simulink model "Solar_Seguidor"  (R2021b)
settings: Solver=ode1  StartTime=0.0  StopTime=inf  FixedStep=25e-6  RelTol=1e-3
PostLoadFcn:
  | %clc; clear all; close all;
  | %%%%%%%%%%%%%%%%%%%%%%%%%%%%%%%%%%%%%%%%%%%%%%%%
  | %%%%%%%%% Solar seguidor de rede %%%%%%%%%%
  | %%%%%%%%%%%%%%%%%%%%%%%%%%%%%%%%%%%%%%%%%%%%%%%%
  | %%%% Nominal Parameters %%%%
  | Pnom = 16e3;                                         % Potencia Nominal
  | Vnom_rms = 210;                                    % V linha rms
  | Vnom_peak = sqrt(2/3)*Vnom_rms;                     % V fase pico
  | FP_min = 1;                                       % Para suporte de reativo
  | Snom = Pnom/FP_min;                                 % Potencia aparente
  | Irms = Pnom/(sqrt(3)*Vnom_rms);                     % Ig rms
  | Inom_peak = Irms*sqrt(2);                           % Ig pico
  | Zbase = Vnom_peak/Inom_peak;                        % Impedancia Base
  | f = 60;                                             % Freq nominal
  | wnom = 2*pi*60;                                     % Freq Ang. nominal
  | m = 0.805;                                            % Indice mod nominal
  | Vdc = 2*(Vnom_peak/m);                              % Vcc
  | Vdc_2 = Vdc/2;                                      % Metade Vcc
  | Kconv = Zbase;                                      % Ganho conversor
  | %%%% Transformer %%%%
  | S_trafo = 250e3;                                      % transformer apparent power
  | Vrms_high = 400;                                   % transformer secondary voltage - Wye connection
  | Vrms_low = 210;                                   % transformer primary voltage - Delta connection
  | N = Vrms_high/Vrms_low;                             % transformation relationship
  | X_pu_trafo = 0.03;                                 % transformer p.u. reactance
  | Zb_trafo_high = ((Vrms_high)^2)/S_trafo;            % secondary base impedance
  | Zb_trafo = ((Vnom_rms)^2)/S_trafo;                  % primary base impedance
  | L_trafo = (X_pu_trafo*Zb_trafo)/wnom;               % primary inductance
  | %%%% LCL Filter Project %%%%
  | fsw = 105*60;%105*60;                                         % switching frequency
  | ripple = 0.05;                                       % current ripple
  | L1 = Vdc/(6*ripple*Inom_peak*fsw);                  % inductor L1
  |  RL1 = 0.005;                                        % L1 resistance
  |  Cbase = 1/(wnom*Kconv);                             % base capacitance
  |  Cf = 0.05*Cbase;                                    % filter capacitor
  | % Calculo do filtro
  | Sbase = 16e3;
  | %Sbase = 200e3*1.12;
  | V_LL = 210;
  | V_LG = 210/sqrt(3);
  | Vbase = V_LG*sqrt(2);
  | Ibase = (Sbase*sqrt(2))/(V_LG*3)*sqrt(3/2);
  | Zbase = (V_LL^2)/Sbase;
  | Rbase = Zbase;
  | Xbase = Zbase;
  | Lbase = Xbase/(2*pi*60);
  | Cbase = 1/(Xbase*2*pi*60);
  | w = 2*pi*60;
  | Q = 70;
  | Lf = 0.15*Lbase;
  | Cf = 0.05*Cbase;
  | fc = 1/(2*pi*sqrt(Lf*Cf));
  | R = (w*Lf)/Q;
  | Lf = L1;
  | R = RL1;
  | ka=0.2;                                             % attenuation factor
  | L2 = (sqrt(1/(ka^2))+1)/(Cf*((2*pi*fsw)^2));        % inductor L2
  | RL2 = 0.005;                                        % L2 resistance
  | w_res = sqrt((L1+L2+L_trafo)/(L1*L2*Cf));           % resonant angular frequency
  | f_res = w_res/(2*pi);                               % resonant frequency
  | Rf = 1/(3*w_res*Cf);                                % filter capacitor resistance
  | %%%%%%%%%%%%%%%%%%%%%%%%
  | %%%% Control Design %%%%
  | %%%%%%%%%%%%%%%%%%%%%%%%
  | %%%% Power Control %%%%
  | Ron = 0.0001;
  | tau_i = 0.5e-3;                                       % tempo de resposta
  | kp_current = (Lf+L_trafo)/tau_i;
  | ki_current = (R+Ron)/tau_i;
  | decouple = (wnom*Lf);
  | kp_current_pu = kp_current/Kconv;                  % Adaptando para pu
  | ki_current_pu = ki_current/Kconv;
  | decouple_pu = (wnom*Lf+(R+Ron))/Kconv;
  | %%%% Dc Link Control %%%%
  | Iext = Pnom/Vdc;
  | Kcc = Vdc/Iext;
  | Sbase = 16e3;
  | C_cc_proj = (Sbase/(2*pi*60*Vdc*Vdc*0.05));
  | 
  | % Controle de tensao
  | a = 3;
  | kp_dc = (C_cc_proj)/(2*a*tau_i);
  | ti_dc = (a^2)*tau_i;
  | ki_dc = kp_dc/ti_dc;
  | kp_dc_pu = (Kcc*C_cc_proj)/(2*a*tau_i);
  | ki_dc_pu = kp_dc_pu/ti_dc;
  | 
  | Ts = 25e-6;
  | 
  | 
  |  Ts_Control=2*Ts;Ts_Power=Ts;
InitFcn:
  | %clc; clear all; close all;
  | %%%%%%%%%%%%%%%%%%%%%%%%%%%%%%%%%%%%%%%%%%%%%%%%
  | %%%%%%%%% Solar seguidor de rede %%%%%%%%%%
  | %%%%%%%%%%%%%%%%%%%%%%%%%%%%%%%%%%%%%%%%%%%%%%%%
  | %%%% Nominal Parameters %%%%
  | Pnom = 16e3;                                         % Potencia Nominal
  | Vnom_rms = 210;                                    % V linha rms
  | Vnom_peak = sqrt(2/3)*Vnom_rms;                     % V fase pico
  | FP_min = 1;                                       % Para suporte de reativo
  | Snom = Pnom/FP_min;                                 % Potencia aparente
  | Irms = Pnom/(sqrt(3)*Vnom_rms);                     % Ig rms
  | Inom_peak = Irms*sqrt(2);                           % Ig pico
  | Zbase = Vnom_peak/Inom_peak;                        % Impedancia Base
  | f = 60;                                             % Freq nominal
  | wnom = 2*pi*60;                                     % Freq Ang. nominal
  | m = 0.805;                                            % Indice mod nominal
  | Vdc = 2*(Vnom_peak/m);                              % Vcc
  | Vdc_2 = Vdc/2;                                      % Metade Vcc
  | Kconv = Zbase;                                      % Ganho conversor
  | %%%% Transformer %%%%
  | S_trafo = 250e3;                                      % transformer apparent power
  | Vrms_high = 400;                                   % transformer secondary voltage - Wye connection
  | Vrms_low = 210;                                   % transformer primary voltage - Delta connection
  | N = Vrms_high/Vrms_low;                             % transformation relationship
  | X_pu_trafo = 0.03;                                 % transformer p.u. reactance
  | Zb_trafo_high = ((Vrms_high)^2)/S_trafo;            % secondary base impedance
  | Zb_trafo = ((Vnom_rms)^2)/S_trafo;                  % primary base impedance
  | L_trafo = (X_pu_trafo*Zb_trafo)/wnom;               % primary inductance
  | %%%% LCL Filter Project %%%%
  | fsw = 105*60;%105*60;                                         % switching frequency
  | ripple = 0.05;                                       % current ripple
  | L1 = Vdc/(6*ripple*Inom_peak*fsw);                  % inductor L1
  |  RL1 = 0.005;                                        % L1 resistance
  |  Cbase = 1/(wnom*Kconv);                             % base capacitance
  |  Cf = 0.05*Cbase;                                    % filter capacitor
  | % Calculo do filtro
  | Sbase = 16e3;
  | %Sbase = 200e3*1.12;
  | V_LL = 210;
  | V_LG = 210/sqrt(3);
  | Vbase = V_LG*sqrt(2);
  | Ibase = (Sbase*sqrt(2))/(V_LG*3)*sqrt(3/2);
  | Zbase = (V_LL^2)/Sbase;
  | Rbase = Zbase;
  | Xbase = Zbase;
  | Lbase = Xbase/(2*pi*60);
  | Cbase = 1/(Xbase*2*pi*60);
  | w = 2*pi*60;
  | Q = 70;
  | Lf = 0.15*Lbase;
  | Cf = 0.05*Cbase;
  | fc = 1/(2*pi*sqrt(Lf*Cf));
  | R = (w*Lf)/Q;
  | Lf = L1;
  | R = RL1;
  | ka=0.2;                                             % attenuation factor
  | L2 = (sqrt(1/(ka^2))+1)/(Cf*((2*pi*fsw)^2));        % inductor L2
  | RL2 = 0.005;                                        % L2 resistance
  | w_res = sqrt((L1+L2+L_trafo)/(L1*L2*Cf));           % resonant angular frequency
  | f_res = w_res/(2*pi);                               % resonant frequency
  | Rf = 1/(3*w_res*Cf);                                % filter capacitor resistance
  | %%%%%%%%%%%%%%%%%%%%%%%%
  | %%%% Control Design %%%%
  | %%%%%%%%%%%%%%%%%%%%%%%%
  | %%%% Power Control %%%%
  | Ron = 0.0001;
  | tau_i = 0.5e-3;                                       % tempo de resposta
  | kp_current = (Lf+L_trafo)/tau_i;
  | ki_current = (R+Ron)/tau_i;
  | decouple = (wnom*Lf);
  | kp_current_pu = kp_current/Kconv;                  % Adaptando para pu
  | ki_current_pu = ki_current/Kconv;
  | decouple_pu = (wnom*Lf+(R+Ron))/Kconv;
  | %%%% Dc Link Control %%%%
  | Iext = Pnom/Vdc;
  | Kcc = Vdc/Iext;
  | Sbase = 16e3;
  | C_cc_proj = (Sbase/(2*pi*60*Vdc*Vdc*0.05));
  | 
  | % Controle de tensao
  | a = 3;
  | kp_dc = (C_cc_proj)/(2*a*tau_i);
  | ti_dc = (a^2)*tau_i;
  | ki_dc = kp_dc/ti_dc;
  | kp_dc_pu = (Kcc*C_cc_proj)/(2*a*tau_i);
  | ki_dc_pu = kp_dc_pu/ti_dc;
  | 
  | Ts = 25e-6;
  | 
  | 
  |  Ts_Control=2*Ts;Ts_Power=Ts;
undefined symbols (not defined in the file): D1, Delta, DIN_2A_Ch00, DiscIntNeverNeededParam, eHS, I, Kp_dc, Left, parameter_set_id, ph, signal1, signal2, signal3, signal4, signal5, signal6, signal7, type, V
libraries: rtlab x11, spsCurrentMeasurementLib x4, spsabctodq0Lib x4, spsThreePhaseVIMeasurementLib x3, spsThreePhaseSeriesRLCBranchLib x3, spsPLL3phLib x3, spsTHDLib x3, artemis x2, spsOnDelayLib x2, spsSeriesRLCBranchLib x2, spsRMSLib x2, slpidlib x2
(part 1 of 2)
settings Model: ARTEMISmethode_block_infos=$$__separator__$$Solar_Seguidor/ARTEMIS Guide1$$__separator__$$  Creator=Lafae  LastModifiedBy=lafae
settings SolverCC: AlgebraicLoopSolver=LineSearch
settings DataIOCC: SaveOutput=off  SaveTime=off  ReturnWorkspaceOutputs=off
settings OptimizationCC: BlockReduction=off  OptimizeBlockIOStorage=off  BufferReuse=off  GlobalBufferReuse=off  ExpressionFolding=off  LocalBlockOutputs=off  OptimizeDataStoreBuffers=off  BusAssignmentInplaceUpdate=off
settings DebuggingCC: AlgebraicLoopMsg=none  MaxConsecutiveZCsMsg=none  MultiTaskDSMMsg=warning  ParameterOverflowMsg=warning  ModelReferenceExtraNoncontSigs=none  SFMachineParentedDataDiag=warning  ArithmeticOperatorsInVariantConditions=warning
settings SFSimCC: CustomCodeUndefinedFunction=UseInterfaceOnly

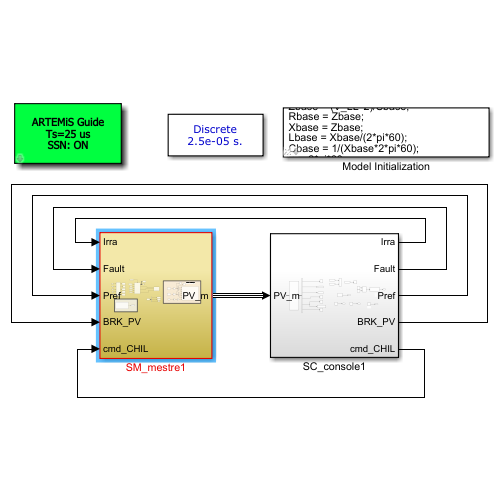
[thumbnail: Simulink's stored preview of the top-level diagram]
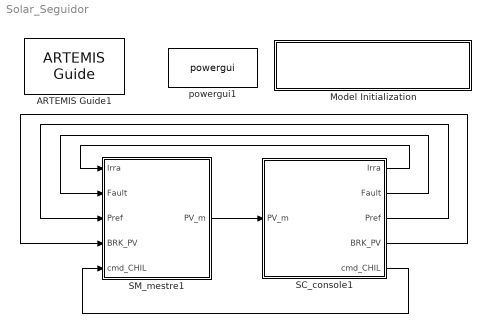
== system Solar_Seguidor ==
  ARTEMIS Guide1 : artemis/ARTEMIS/ARTEMIS Guide  Tag=art7.5  Description=New ARTEMiS block v 7.5b (R2015b+)  lock=on  Ts=Ts  ssn=on  opt=art5  dyna=off  nb_perm=4  RT_fullcomp=off  ssn_itvc=off  ssn_ivic=off  ssn_ext=off  ssn_solver=Art5  iter_type=iSWITCH and iMOV only (default)  ssn_ImpulseLoopBlockedStateUpdate=5  ssn_mov_iter_number=5  ssn_switch_iter_number=3  ssn_lu_or_ldlt=LU (more robust)  ssn_nib_type_verify=on  ssn_use_lu=on  ssn_use_ldlt=off  ssn_impulse=on  ssn_quasimpulse=off  ssn_impulse_loop=5  paraExtinctionThy=off  Thy_Impulse=on  dtc=Off  dtc_opt=normal  ao=off  simtype=off  ct_mac=off  lin_mov=off  lsp=[0.001 2]  spike_skip=Disabled  dtc_extra=1  dtc_sws=normal  dtc_pied=0.5  SPSRulesBlock=SPSRules  tre=off  ctmm=off  LF=off  dpl_type=ARTEMiS DPL  rlc_type=off  custom_type=off  para=on  ssn_full_iteration=off  ssn_init_cond=block only
  Model Initialization : Subsystem  AncestorBlock=artemis/Tools /Misc/Model Initialization  mask(Model Functions){InitFcnX=|, prel=off, posl=on, inif=on, strf=off}
      mask InitFcnX=|
      | %clc; clear all; close all;
      | %%%%%%%%%%%%%%%%%%%%%%%%%%%%%%%%%%%%%%%%%%%%%%%%
      | %%%%%%%%% Solar seguidor de rede %%%%%%%%%%
      | %%%%%%%%%%%%%%%%%%%%%%%%%%%%%%%%%%%%%%%%%%%%%%%%
      | %%%% Nominal Parameters %%%%
      | Pnom = 16e3;                                         % Potencia Nominal
      | Vnom_rms = 210;                                    % V linha rms
      | Vnom_peak = sqrt(2/3)*Vnom_rms;                     % V fase pico
      | FP_min = 1;                                       % Para suporte de reativo
      | Snom = Pnom/FP_min;                                 % Potencia aparente
      | Irms = Pnom/(sqrt(3)*Vnom_rms);                     % Ig rms
      | Inom_peak = Irms*sqrt(2);                           % Ig pico
      | Zbase = Vnom_peak/Inom_peak;                        % Impedancia Base
      | f = 60;                                             % Freq nominal
      | wnom = 2*pi*60;                                     % Freq Ang. nominal
      | m = 0.805;                                            % Indice mod nominal
      | Vdc = 2*(Vnom_peak/m);                              % Vcc
      | Vdc_2 = Vdc/2;                                      % Metade Vcc
      | Kconv = Zbase;                                      % Ganho conversor
      | %%%% Transformer %%%%
      | S_trafo = 250e3;                                      % transformer apparent power
      | Vrms_high = 400;                                   % transformer secondary voltage - Wye connection
      | Vrms_low = 210;                                   % transformer primary voltage - Delta connection
      | N = Vrms_high/Vrms_low;                             % transformation relationship
      | X_pu_trafo = 0.03;                                 % transformer p.u. reactance
      | Zb_trafo_high = ((Vrms_high)^2)/S_trafo;            % secondary base impedance
      | Zb_trafo = ((Vnom_rms)^2)/S_trafo;                  % primary base impedance
      | L_trafo = (X_pu_trafo*Zb_trafo)/wnom;               % primary inductance
      | %%%% LCL Filter Project %%%%
      | fsw = 105*60;%105*60;                                         % switching frequency
      | ripple = 0.05;                                       % current ripple
      | L1 = Vdc/(6*ripple*Inom_peak*fsw);                  % inductor L1
      |  RL1 = 0.005;                                        % L1 resistance
      |  Cbase = 1/(wnom*Kconv);                             % base capacitance
      |  Cf = 0.05*Cbase;                                    % filter capacitor
      | % Calculo do filtro
      | Sbase = 16e3;
      | %Sbase = 200e3*1.12;
      | V_LL = 210;
      | V_LG = 210/sqrt(3);
      | Vbase = V_LG*sqrt(2);
      | Ibase = (Sbase*sqrt(2))/(V_LG*3)*sqrt(3/2);
      | Zbase = (V_LL^2)/Sbase;
      | Rbase = Zbase;
      | Xbase = Zbase;
      | Lbase = Xbase/(2*pi*60);
      | Cbase = 1/(Xbase*2*pi*60);
      | w = 2*pi*60;
      | Q = 70;
      | Lf = 0.15*Lbase;
      | Cf = 0.05*Cbase;
      | fc = 1/(2*pi*sqrt(Lf*Cf));
      | R = (w*Lf)/Q;
      | Lf = L1;
      | R = RL1;
      | ka=0.2;                                             % attenuation factor
      | L2 = (sqrt(1/(ka^2))+1)/(Cf*((2*pi*fsw)^2));        % inductor L2
      | RL2 = 0.005;                                        % L2 resistance
      | w_res = sqrt((L1+L2+L_trafo)/(L1*L2*Cf));           % resonant angular frequency
      | f_res = w_res/(2*pi);                               % resonant frequency
      | Rf = 1/(3*w_res*Cf);                                % filter capacitor resistance
      | %%%%%%%%%%%%%%%%%%%%%%%%
      | %%%% Control Design %%%%
      | %%%%%%%%%%%%%%%%%%%%%%%%
      | %%%% Power Control %%%%
      | Ron = 0.0001;
      | tau_i = 0.5e-3;                                       % tempo de resposta
      | kp_current = (Lf+L_trafo)/tau_i;
      | ki_current = (R+Ron)/tau_i;
      | decouple = (wnom*Lf);
      | kp_current_pu = kp_current/Kconv;                  % Adaptando para pu
      | ki_current_pu = ki_current/Kconv;
      | decouple_pu = (wnom*Lf+(R+Ron))/Kconv;
      | %%%% Dc Link Control %%%%
      | Iext = Pnom/Vdc;
      | Kcc = Vdc/Iext;
      | Sbase = 16e3;
      | C_cc_proj = (Sbase/(2*pi*60*Vdc*Vdc*0.05));
      |
      | % Controle de tensao
      | a = 3;
      | kp_dc = (C_cc_proj)/(2*a*tau_i);
      | ti_dc = (a^2)*tau_i;
      | ki_dc = kp_dc/ti_dc;
      | kp_dc_pu = (Kcc*C_cc_proj)/(2*a*tau_i);
      | ki_dc_pu = kp_dc_pu/ti_dc;
      |
      | Ts = 25e-6;
      |
      |
      |  Ts_Control=2*Ts;Ts_Power=Ts;
      mask prompts: InitFcnX "Initialisation"; prel "Preload Function"; posl "PostLoad Function"; inif "InitFcn"; strf "StartFcn"
      mask init:
      | currentBlock = gcb;
      | root = bdroot(currentBlock);
      | 
      | if ~strcmp(get_param(root,'BlockDiagramType'),'library')
      |     if prel==1
      |         set_param(root, 'PreLoadFcn', InitFcnX);
      |     else
      |         set_param(root, 'PreLoadFcn', '');
      |     end
      |     if inif==1
      |         set_param(root, 'InitFcn', InitFcnX);
      |     else
      |         set_param(root, 'InitFcn', '');
      |     end
      |     if strf==1
      |         set_param(root, 'StartFcn', InitFcnX);
      |     else
      |         set_param(root, 'StartFcn', '');
      |     end
      |     if posl==1
      |         set_param(root, 'PostLoadFcn', InitFcnX);
      |     else
      |         set_param(root, 'PostLoadFcn', '');
      |     end
      | end
      | 
      | pos = get_param(currentBlock, 'Position');
      | width = pos(3) - pos(1); height = pos(4) - pos(2);
      | txt = [ upper(root) '\n' '- InitFcn. . . . . '  get_param(root, 'InitFcn') ];
      settings: CopyFcn=set_param(gcb,'LinkStatus','inactive')
      mask Display: text(5, height*0.5, txt, 'horizontalAlignment', 'left', 'verticalAlignment', 'middle') ;
  SC_console1 : Subsystem
  SM_mestre1 : Subsystem
  powergui1 : spspowerguiLib/powergui  Priority=1  SimulationMode=Discrete  SampleTime=Ts  frequency=60  Iterations=50  frequencyindice=0  Pbase=100e6  ErrMax=1e-4  UnitsV=kV  UnitsW=MW  buscounter=0  FunctionMessages=off  echomessages=off  EnableUseOfTLC=off  CurrentSourceSwitches=off  DisableSnubberDevices=off  DisableRonSwitches=off  DisableVfSwitches=off  DisplayEquations=off  AutomaticDiscreteSolvers=off  SolverType=Tustin/Backward Euler (TBE)  Interpol=off  ExternalGateDelay=off  methode=off  Ts=0  x0status=blocks  SPID=off  SwTol=0  HookPort=off  NonlinearTolerance=0  nMaxIteration=15  ContinueOnMaxIteration=off  RestoreLinks=warning  ResistiveCurrentMeasurement=off  Frange=[0:2:500]  Ylog=off  Xlog=on  ShowGrid=off  save=off  variable=ZData  structure=0  ZoomFFT=on  StartTime=0.0  cycles=1  DisplayStyle=1  fundamental=60  FreqAxis=off  MaxFrequency=1000  frequencyindicesteady=1  RmsSteady=1  display=off
  wires:
  SM_mestre1/1(PV_m) -> SC_console1/1(PV_m)
  SC_console1/1(Irra) -> SM_mestre1/1(Irra)
  SC_console1/2(Fault) -> SM_mestre1/2(Fault)
  SC_console1/3(Pref) -> SM_mestre1/3(Pref)
  SC_console1/4(BRK_PV) -> SM_mestre1/4(BRK_PV)
  SC_console1/5(cmd_CHIL) -> SM_mestre1/5(cmd_CHIL)

== system Solar_Seguidor/Model Initialization ==

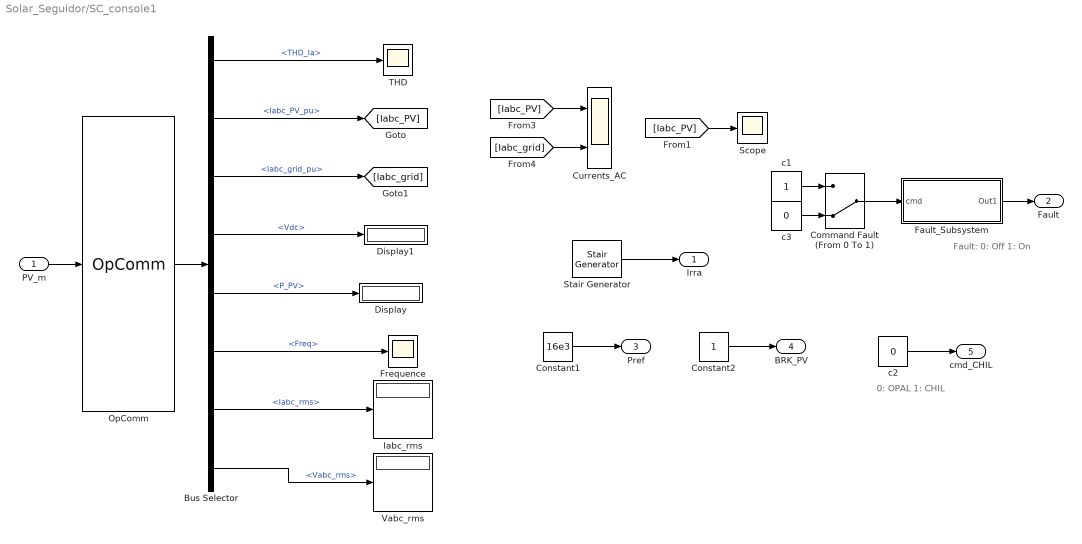
== system Solar_Seguidor/SC_console1 ==
  note: Fault:
      | 0: Off
      | 1: On
  note: 0: OPAL
      | 1: CHIL
  PV_m : Inport
  Bus Selector : BusSelector  OutputSignals=THD_Ia,Iabc_PV_pu,Iabc_grid_pu,Vdc,P_PV,Freq,Iabc_rms,Vabc_rms
  Command Fault (From 0 To 1) : ManualSwitch  CurrentSetting=0
  Constant1 : Constant  Value=16e3
  Constant2 : Constant
  Currents_AC : Scope  NumInputPorts=2
  Display : Display
  Display1 : Display
  Fault_Subsystem : Subsystem
  Frequence : Scope
  Iabc_rms : Display
  OpComm : rtlab/OpComm  nbport=1  groupe_acq=1  subsys_rate=0  st=0  Synchronization=on  Interpolation=on  Threshold=1.0  Missed_Data=off  Sim_Time=off  Samples=off  dynSigOut=off  from_console=0  warning_done=off  writeOpCommFile=off  Offset=off
      settings: SourceProductName=RT-LAB
  Scope : Scope
  Stair Generator : spsStairGeneratorLib/Stair Generator  t=[0, 1, 3, 5,7]  e=[10, 4, 7.5, 10,10]*1e2  Ts=0
  THD : Scope
  Vabc_rms : Display
  c1 : Constant
  c2 : Constant  Value=0
  c3 : Constant  Value=0
  Irra : Outport
  Fault : Outport  Port=2
  Pref : Outport  Port=3
  BRK_PV : Outport  Port=4
  cmd_CHIL : Outport  Port=5
  wires:
  [Iabc_PV] -> Currents_AC/1
  [Iabc_grid] -> Currents_AC/2
  PV_m/1 -> OpComm/1
  Bus Selector/2 -> [Iabc_PV]  "<Iabc_PV_pu>"
  Stair Generator/1 -> Irra/1
  Fault_Subsystem/1(Out1) -> Fault/1
  c1/1 -> Command Fault (From 0 To 1)/1
  c3/1 -> Command Fault (From 0 To 1)/2
  Command Fault (From 0 To 1)/1 -> Fault_Subsystem/1(cmd)
  Constant1/1 -> Pref/1
  [Iabc_PV] -> Scope/1
  OpComm/1 -> Bus Selector/1
  Bus Selector/1 -> THD/1  "<THD_Ia>"
  Bus Selector/3 -> [Iabc_grid]  "<Iabc_grid_pu>"
  Bus Selector/4 -> Display1/1  "<Vdc>"
  Bus Selector/5 -> Display/1  "<P_PV>"
  Bus Selector/6 -> Frequence/1  "<Freq>"
  Constant2/1 -> BRK_PV/1
  c2/1 -> cmd_CHIL/1
  Bus Selector/7 -> Iabc_rms/1  "<Iabc_rms>"
  Bus Selector/8 -> Vabc_rms/1  "<Vabc_rms>"

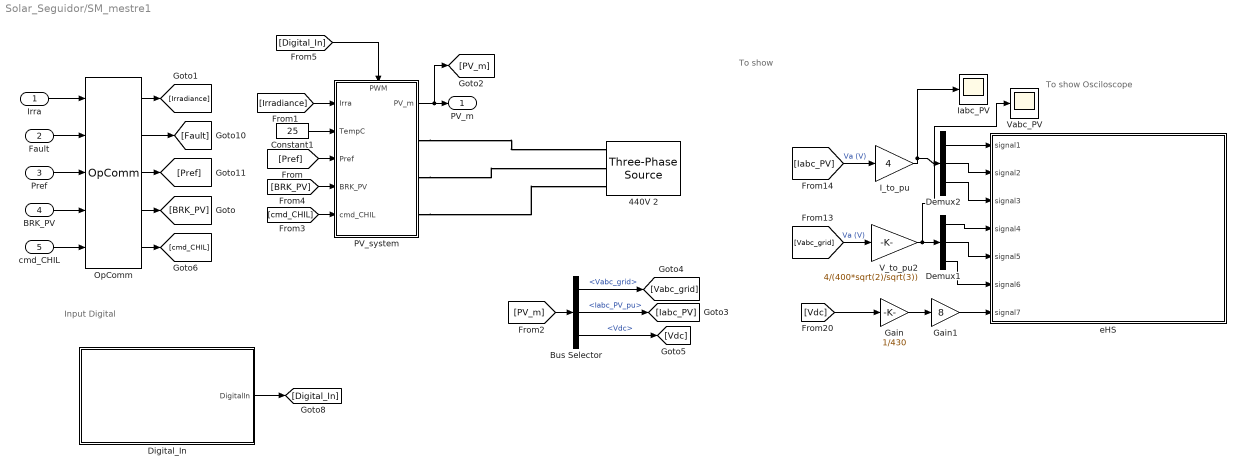
== system Solar_Seguidor/SM_mestre1 ==
  note: To show Osciloscope
  note: To show
  note: Input Digital
  Irra : Inport
  Fault : Inport  Port=2
  Pref : Inport  Port=3
  BRK_PV : Inport  Port=4
  cmd_CHIL : Inport  Port=5
  440V 2 : spsThreePhaseSourceLib/Three-Phase Source  InternalConnection=Yg  VoltagePhases=off  Voltage=400  PhaseAngle=0  Voltage_phases=[25e3 25e3 25e3]/sqrt(3)  PhaseAngles_phases=[0 -120 +120]  Frequency=60  NonIdealSource=on  SpecifyImpedance=on  Resistance=0.8929  Inductance=16.58e-3  ShortCircuitLevel=2500e6  BaseVoltage=400  XRratio=7  BusType=swing  Pref=0  Qref=0  Prefabc=[10e3, 10e3, 10e3]  Qrefabc=[0, 0, 0]  Qmin=-inf  Qmax=inf
  Bus Selector : BusSelector  OutputSignals=Vabc_grid,Iabc_PV_pu,Vdc
  Constant1 : Constant  Value=25
  Demux1 : Demux  Outputs=3
  Demux2 : Demux  Outputs=3
  Digital_In : Subsystem
  Gain : Gain  Gain=1/430
  Gain1 : Gain  Gain=8
  I_to_pu : Gain  Gain=4  SaturateOnIntegerOverflow=on  OutDataTypeStr=Inherit: Same as input  ParamDataTypeStr=Inherit: Same as input
  Iabc_PV : Scope
  OpComm : rtlab/OpComm  nbport=5  groupe_acq=1  subsys_rate=0  st=0  Synchronization=on  Interpolation=on  Threshold=1.0  Missed_Data=off  Sim_Time=off  Samples=off  dynSigOut=off  from_console=1  warning_done=off  writeOpCommFile=off  Offset=off
      settings: SourceProductName=RT-LAB
  PV_system : Subsystem
      settings: PortSchema="{\"entries\":[{\"content\":{\"sides\":[{\"content\":{\"connectorIds\":[\"In1\",\"In2\",\"In3\",\"In4\",\"In5\"]},\"type\":\"ConnectorPlacement.EquallySpacedRectSide\",\"uuid\":\"f9680090-159c-44c1-a82d-3351337b351d\"},{\"content\":{\"connectorIds\":[\"Out1\",\"RConn1\",\"RConn2\",\"RConn3\"],\"side\":\"RIGHT\"},\"type\":\"ConnectorPlacement.EquallySpacedRectSide\",\"uuid\":\"a8520c85-fa09-4516-b22e-d1ac2b1a084c\"},{\"content\":{\"connectorIds\":[\"In6\"],\"side\":\"TOP\"},\"type\":\"ConnectorPlacement.EquallySpacedRectSide\",\"uuid\":\"db03fa81-c690-4cf1-8b9d-a41123e25ef4\"}]},\"type\":\"ConnectorPlacement.EquallySpacedConnector\",\"uuid\":\"3e739a15-12b1-4a95-8158-3bf7b6288ced\"}],\"packageUris\":[\"http://schema.mathworks.com/mf0/Connector/R2020b\"],\"version\":\"1.0\"}"
  V_to_pu2 : Gain  Gain=4/(400*sqrt(2)/sqrt(3))  SaturateOnIntegerOverflow=on  OutDataTypeStr=Inherit: Same as input  ParamDataTypeStr=Inherit: Same as input
  Vabc_PV : Scope
  eHS : Subsystem  mask{ModelsList=Test_IO - v1 (2022-07-08T13:54:53.656356), Timestamp=Circuit loaded on 06-Jun-2023 21:43:07, ShowInLibBrowser=on, SourceSetList=Internal, ActiveSetList=(0) Default set}
      mask help:
      | This block allows the configuration and the control of an FPGA-based circuit simulation using eHS Power Electronics toolbox.
      | The circuit is edited using OPAL-RT Schematic Editor.
      settings: CopyFcn=set_param(gcb,'LinkStatus','none');  OpenFcn=ehsGen4BlockLastModelLoadedCb(gcb)
      mask Help: web(['file:///' getenv('EFPGASIM_ROOT') '/Docs/html/eFPGAsim/efs_eHSgen4_SE.html']);
      mask TypeOptions ModelsList: Aout_16ch - v1 (2023-04-29T00:08:17.716757) | Aout_16ch - v1 (2022-05-12T13:44:17.536927) | Aout_16ch - v1 (2023-04-19T15:00:26.919337) | Aout_16ch - v1 (2023-04-19T16:51:28.908908) | Boost2lvl_OP4200 - v1 | Boost2lvl_OP5700 - v1 (2023-02-10T10:43:47.36416) | Boost2lvl_OP5700 - v1 (2022-11-12T13:44:36.956611) | Boost2lvl_OP5700 - v1 (2023-05-08T22:29:57.421012) | Boost2lvl_OP5700 - v1 (2023-05-18T10:01:41.903526) | Boost2lvl_OP5700 - v1 (2022-11-12T11:44:54.058648) | Boost2lvl_OP5700 - v1 (2022-11-16T17:55:25.832987) | Boost2lvl_OP5700 - v1 (2023-06-01T11:05:48.96312) | Boost2lvl_OP5700 - v1 (2023-04-17T17:49:19.968569) | Boost2lvl_OP5700 - v1 (2023-05-30T16:08:17.821314) | Boost2lvl_OP5700 - v1 (2022-11-24T13:51:49.960507) | Boost2lvl_OP5700 - v1 (2023-04-14T14:44:54.884125) | Boost2lvl_OP5700 - v1 (2023-02-02T11:36:19.810304) | Boost2lvl_OP5700 - v1 (2022-11-12T12:53:45.024286) | Boost2lvl_OP5700 - v1 (2023-05-05T11:44:28.956217) | DFIM_OP5700 - v1 | Hands_on_No1_FPGA - v1 | Hands_on_No2_FPGA - v1 | Hands_on_No3_FPGA - v1 (2023-05-17T11:33:17.751604) | Hands_on_No3_FPGA - v1 (2023-05-09T21:46:39.434647) | Hands_on_No4_FPGA - v1 (2023-05-17T21:24:20.423955) | Hands_on_No4_FPGA - v1 (2023-05-09T22:05:23.628908) | Inverter_FPGA - v1 | NPC Inverter - OP5607 - v1 (2022-11-12T14:04:00.927404) | NPC Inverter - OP5607 - v1 (2022-11-12T12:55:50.543618) | PMSMDriveOP5707 - v1 (2022-05-19T14:22:57.093341) | PMSMDriveOP5707 - v1 (2022-05-19T14:21:06.997063) | SCIM_OP5700 - v1 (2022-05-19T14:45:26.789519) | SCIM_OP5700 - v1 (2022-11-12T14:00:15.548565) | SCIM_OP5700 - v1 (2022-11-14T13:40:01.1266) | Test_coSimulation - v1 | Test_FPGA_Andre - v1 (2023-05-08T22:34:34.161353) | Test_FPGA_Andre - v1 (2023-05-08T17:39:09.275335) | Test_FPGA_Andre - v1 (2023-05-05T09:27:35.819562) | Test_IO - v1 (2023-06-06T10:23:50.206639) | Test_IO - v1 (2022-10-12T12:22:10.646782) | Test_IO - v1 (2022-07-08T13:54:53.656356) | Test_IO - v1 (2023-05-24T23:06:22.353175)
      mask Callback ModelsList: ehsGen4BlockFillModelListCb(gcb);
      mask TypeOptions SourceSetList: Internal | External
      mask Callback SourceSetList: ehsGen4BlockParamSetSourceCb(gcb);
      mask TypeOptions ActiveSetList: (0) Default set
      mask DialogControl ParameterGroupVar Prompt: Circuit
      mask DialogControl ModelName Prompt: Name
      mask DialogControl Refresh Callback: ehsGen4BlockFillModelListCb(gcb);
      mask DialogControl Edit Prompt: Edit
      mask DialogControl Edit Callback: ehsGen4BlockEditModelCb(gcb);
      mask DialogControl CreateNew Prompt: Create new
      mask DialogControl CreateNew Callback: ehsGen4BlockCreateModelCb(gcb);
      mask DialogControl Load Prompt: Load circuit
      mask DialogControl Load Callback: ehsGen4BlockLoadModelCb(gcb);
      mask DialogControl ErrorLink Prompt: More configuration details
      mask DialogControl ErrorLink Callback: ehsGen4BlockNotificationPopupCb(gcb);
      mask DialogControl ParameterSetGroup Prompt: Parameter set
      mask DialogControl Source Prompt: Source
      mask DialogControl ActiveSet Prompt: Active set
      mask DialogControl Uuid Prompt: e434fd9d-0952-4cea-a2b3-27fd494b0346
      mask DialogControl LastModelLoaded Prompt: Test_IO - v1 (2022-07-08T13:54:53.656356)
      mask Display:
      | fprintf('eHS\n\n')
      | fprintf(ehsGen4BlockGetLastModelLoaded(gcb))
      | ehsGen4BlockUpdateConstantBlockCb(gcb)
      | ehsGen4BlockAddLabel
  PV_m : Outport
  wires:
  Irra/1 -> OpComm/1
  Fault/1 -> OpComm/2
  OpComm/2 -> [Fault]
  Pref/1 -> OpComm/3
  OpComm/3 -> [Pref]
  Constant1/1 -> PV_system/2(TempC)
  PV_system/1(PV_m) -> [PV_m], PV_m/1
  [Pref] -> PV_system/3(Pref)
  OpComm/1 -> [Irradiance]
  [Irradiance] -> PV_system/1(Irra)
  [BRK_PV] -> PV_system/4(BRK_PV)
  OpComm/4 -> [BRK_PV]
  BRK_PV/1 -> OpComm/4
  Demux2/3 -> eHS/3(signal3)
  Gain1/1 -> eHS/7(signal7)
  Demux2/2 -> eHS/2(signal2)
  [Vdc] -> Gain/1
  [Iabc_PV] -> I_to_pu/1  "Va (V)"
  I_to_pu/1 -> Iabc_PV/1, Demux2/1
  Gain/1 -> Gain1/1
  Demux1/3 -> eHS/6(signal6)
  Demux2/1 -> eHS/1(signal1)
  Demux1/1 -> eHS/4(signal4)
  [Vabc_grid] -> V_to_pu2/1  "Va (V)"
  Demux1/2 -> eHS/5(signal5)
  [PV_m] -> Bus Selector/1
  Bus Selector/2 -> [Iabc_PV]  "<Iabc_PV_pu>"
  Bus Selector/1 -> [Vabc_grid]  "<Vabc_grid>"
  Bus Selector/3 -> [Vdc]  "<Vdc>"
  V_to_pu2/1 -> Vabc_PV/1, Demux1/1
  cmd_CHIL/1 -> OpComm/5
  OpComm/5 -> [cmd_CHIL]
  [cmd_CHIL] -> PV_system/5(cmd_CHIL)
  Digital_In/1(DigitalIn) -> [Digital_In]
  [Digital_In] -> PV_system/6(PWM)
  connections:
  PV_system/RConn1 -- 440V 2/RConn1
  PV_system/RConn2 -- 440V 2/RConn2
  PV_system/RConn3 -- 440V 2/RConn3

== system Solar_Seguidor/SC_console1/Fault_Subsystem ==
  note: Note: This is the control of the three-phase fault.
  cmd : Inport
  Constant1 : Constant  Value=0
  On Delay : spsOnDelayLib/On Delay  DelayType=On delay  delay=5/60  ic=0  Ts=0
      settings: SourceProductBaseCode=PS
  Scope : Scope
  Switch : Switch  Criteria=u2 > Threshold
  Out1 : Outport
  wires:
  Switch/1 -> Scope/1, Out1/1
  Constant1/1 -> Switch/1
  On Delay/1 -> Switch/2
  cmd/1 -> Switch/3, On Delay/1

== system Solar_Seguidor/SM_mestre1/Digital_In ==
  Bus Creator : BusCreator  Inputs=6
  Cast To Double : DataTypeConversion  OutDataTypeStr=double
  Cast To Double1 : DataTypeConversion  OutDataTypeStr=double
  Cast To Double2 : DataTypeConversion  OutDataTypeStr=double
  DIN_2A_Ch00-07 : rtlab/OpInput  identifier_use=[]  identifier_hide=DIN_2A_Ch00-07  nb_parents_identifier=0  passthrough=off  init_value=zeros(1,8)  value_type=double  create_alias=on
      settings: SourceProductName=RT-LAB
  Demux : Demux  Outputs=8
  NOT : Logic  Operator=NOT  IconShape=distinctive  AllPortsSameDT=off  OutDataTypeStr=boolean
  NOT1 : Logic  Operator=NOT  IconShape=distinctive  AllPortsSameDT=off  OutDataTypeStr=boolean
  NOT2 : Logic  Operator=NOT  IconShape=distinctive  AllPortsSameDT=off  OutDataTypeStr=boolean
  Terminator{,1..4} (5 alike) : Terminator
  DigitalIn : Outport
  wires:
  DIN_2A_Ch00-07/1 -> Demux/1  "DigitalIn_2A_Ch00-07"
  Demux/7 -> Terminator/1
  Demux/6 -> Terminator1/1
  Demux/5 -> Terminator2/1
  Demux/4 -> Terminator3/1
  Demux/1 -> Bus Creator/1, NOT/1  "S1"
  Demux/2 -> Bus Creator/3, NOT1/1  "S3"
  Demux/3 -> Bus Creator/5, NOT2/1  "S5"
  NOT/1 -> Cast To Double/1  "S2"
  NOT1/1 -> Cast To Double1/1  "S4"
  Bus Creator/1 -> DigitalIn/1
  NOT2/1 -> Cast To Double2/1  "S6"
  Cast To Double/1 -> Bus Creator/2  "S2"
  Cast To Double1/1 -> Bus Creator/4  "S4"
  Cast To Double2/1 -> Bus Creator/6  "S6"
  Demux/8 -> Terminator4/1

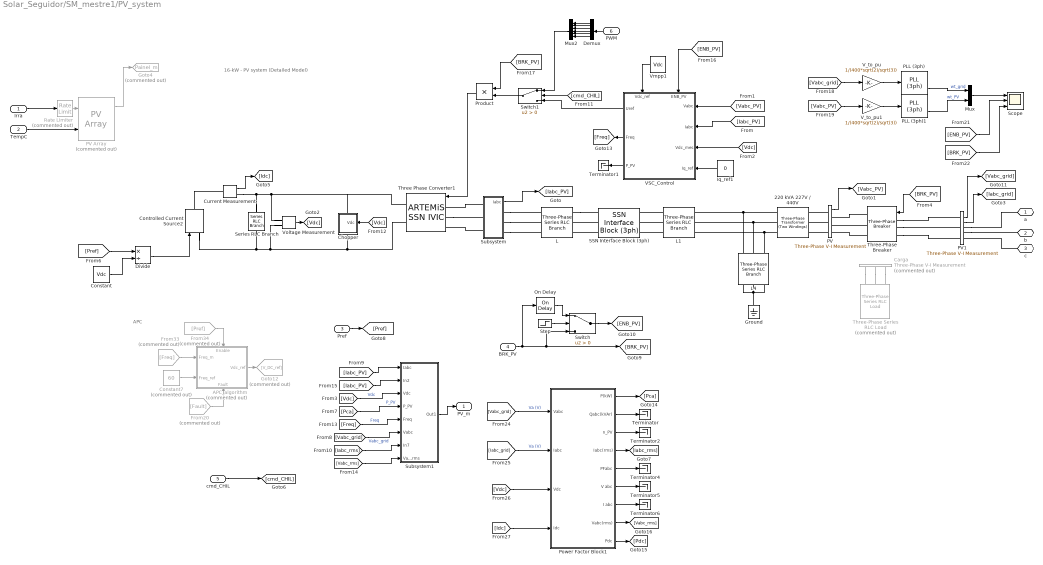
== system Solar_Seguidor/SM_mestre1/PV_system ==
  note: 16-kW - PV system (Detailed Model)
  note: APC
  Irra : Inport
  TempC : Inport  Port=2
  Pref : Inport  Port=3
  BRK_PV : Inport  Port=4
  cmd_CHIL : Inport  Port=5
  PWM : Inport  Port=6
  220 kVA 227V / 440V : spsThreePhaseTransformerTwoWindingsLib/Three-Phase Transformer (Two Windings)  Winding1Connection=Yg  Winding2Connection=Delta (D1)  CoreType=Three single-phase transformers  SetSaturation=off  Hysteresis=off  DataFile='hysteresis'  SetInitialFlux=off  Measurements=None  UNITS=pu  NominalPower=[220e3 , 60 ]  Winding1=[400 , 0.001 , 0.03 ]  Winding2=[210 , 0.001 , 0.03 ]  Rm=500  Lm=500  L0=0.5  Saturation=[ 0,0 ; 0.0024,1.2 ; 1.0,1.52 ]  InitialFluxes=[ 0.8 , -0.8 , 0.7 ]  BreakLoop=off  DiscreteSolver=Trapezoidal iterative  DataType=off  TransfoNumber=0
  APC_algorithm : Subsystem  Commented=on
      settings: PortSchema="{\"entries\":[{\"content\":{\"sides\":[{\"content\":{\"connectorIds\":[\"In1\",\"In2\"]},\"type\":\"ConnectorPlacement.EquallySpacedRectSide\",\"uuid\":\"40656380-5e11-4201-a16e-0974ed2bdfa3\"},{\"content\":{\"connectorIds\":[\"Out1\"],\"side\":\"RIGHT\"},\"type\":\"ConnectorPlacement.EquallySpacedRectSide\",\"uuid\":\"b720f4a2-445d-4911-b95b-a16e7ba2ef90\"},{\"content\":{\"connectorIds\":[\"In3\"],\"side\":\"TOP\"},\"type\":\"ConnectorPlacement.EquallySpacedRectSide\",\"uuid\":\"61735eee-8c6f-4b86-833d-6912c6cea25a\"},{\"content\":{\"connectorIds\":[\"In4\"],\"side\":\"BOTTOM\"},\"type\":\"ConnectorPlacement.EquallySpacedRectSide\",\"uuid\":\"0dbf41d0-9732-4713-8148-d584ab86d8ba\"},{\"content\":{\"connectorIds\":[],\"side\":\"HIDDEN\"},\"type\":\"ConnectorPlacement.EquallySpacedRectSide\",\"uuid\":\"d2c68c6b-be31-4766-a941-11238d66741c\"}]},\"type\":\"ConnectorPlacement.EquallySpacedConnector\",\"uuid\":\"e0287d46-a6c7-46a5-bd63-f4e94fb98690\"}],\"packageUris\":[\"http://schema.mathworks.com/mf0/Connector/R2020b\"],\"version\":\"1.0\"}"
  Carga : spsThreePhaseVIMeasurementLib/Three-Phase V-I Measurement  Commented=on  VoltageMeasurement=phase-to-ground  SetLabelV=on  LabelV=Vcarga  Vpu=off  VpuLL=off  CurrentMeasurement=yes  SetLabelI=on  LabelI=Icarga  Ipu=off  Pbase=100e6  Vbase=500e3  OutputType=Magnitude  PhasorSimulation=off  PSBequivalent=0
  Chopper : Subsystem
      settings: PortSchema="{\"entries\":[{\"content\":{\"sides\":[{\"content\":{\"connectorIds\":[\"In1\"]},\"type\":\"ConnectorPlacement.EquallySpacedRectSide\",\"uuid\":\"afae15e8-9223-41bd-a608-c674f09af6e2\"},{\"content\":{\"connectorIds\":[],\"side\":\"RIGHT\"},\"type\":\"ConnectorPlacement.EquallySpacedRectSide\",\"uuid\":\"cb9b7558-c628-44d0-80da-cf5d18275618\"},{\"content\":{\"connectorIds\":[\"LConn1\"],\"side\":\"TOP\"},\"type\":\"ConnectorPlacement.EquallySpacedRectSide\",\"uuid\":\"c88d4dd8-d7d7-4e14-b7a4-0eec64926e8d\"},{\"content\":{\"connectorIds\":[\"RConn1\"],\"side\":\"BOTTOM\"},\"type\":\"ConnectorPlacement.EquallySpacedRectSide\",\"uuid\":\"ab8565b7-86d8-4527-bc77-6958d129015e\"},{\"content\":{\"connectorIds\":[],\"side\":\"HIDDEN\"},\"type\":\"ConnectorPlacement.EquallySpacedRectSide\",\"uuid\":\"6e2c338e-67f9-4124-b98b-378f1e893452\"}]},\"type\":\"ConnectorPlacement.EquallySpacedConnector\",\"uuid\":\"e63e5afb-0df2-495a-a26c-49d94a1ed139\"}],\"packageUris\":[\"http://schema.mathworks.com/mf0/Connector/R2020b\"],\"version\":\"1.0\"}"
  Constant : Constant  Value=Vdc
  Constant7 : Constant  Commented=on  Value=60
  Controlled Current Source2 : spsControlledCurrentSourceLib/Controlled Current Source  Initialize=on  Source_Type=DC  Amplitude=0  Phase=0  Frequency=0  Measurements=None
  Current Measurement : spsCurrentMeasurementLib/Current Measurement  PhasorSimulation=off  OutputType=Complex  PSBequivalent=0
  Demux : Demux  Outputs=6
  Divide : Product  Inputs=*/
  From20 : From  Commented=on  GotoTag=Fault
  From33 : From  Commented=on  GotoTag=Freq
  From34 : From  Commented=on  GotoTag=Pref
  Goto12 : Goto  Commented=on  GotoTag=V_DC_ref
  Goto4 : Goto  Commented=on  GotoTag=Painel_m  TagVisibility=global
  Ground : spsGroundLib/Ground  LConnTagsString=a
  Iq_ref1 : Constant  Value=0
  L : spsThreePhaseSeriesRLCBranchLib/Three-Phase Series RLC Branch  LConnTagsString=A|B|C  RConnTagsString=A|B|C  BranchType=R  Resistance=R  Inductance=500e-6/2  Capacitance=inf  Measurements=None
  L1 : spsThreePhaseSeriesRLCBranchLib/Three-Phase Series RLC Branch  LConnTagsString=A|B|C  RConnTagsString=A|B|C  BranchType=L  Resistance=500e-6*377/50/2  Inductance=Lf  Capacitance=inf  Measurements=None
  L4 : spsThreePhaseSeriesRLCBranchLib/Three-Phase Series RLC Branch  LConnTagsString=A|B|C  RConnTagsString=A|B|C  BranchType=R  Resistance=1e8  Inductance=Lf  Capacitance=Cf  Measurements=None
  Mux : Mux  Inputs=2
  Mux2 : Mux  Inputs=6
  On Delay : spsOnDelayLib/On Delay  DelayType=On delay  delay=134e-3  ic=0  Ts=0
      settings: SourceProductBaseCode=PS
  PLL (3ph) : spsPLL3phLib/PLL (3ph)  Fmin=45  Par_Init="[-0.57  60]"  ParK=[180, 3200, 1]  TcD=Ts_Control  MaxRateChangeFreq=12  FilterCutOffFreq=25  Ts=Ts_Control  AGC=on
  PLL (3ph)1 : spsPLL3phLib/PLL (3ph)  Fmin=45  Par_Init="[-0.57  60]"  ParK=[180, 3200, 1]  TcD=Ts_Control  MaxRateChangeFreq=12  FilterCutOffFreq=25  Ts=Ts_Control  AGC=on
  PV : spsThreePhaseVIMeasurementLib/Three-Phase V-I Measurement  VoltageMeasurement=phase-to-ground  SetLabelV=off  LabelV=Vabc_grid  Vpu=off  VpuLL=off  CurrentMeasurement=no  SetLabelI=off  LabelI=Iabc_grid  Ipu=off  Pbase=100e6  Vbase=500e3  OutputType=Magnitude  PhasorSimulation=off  PSBequivalent=0
  PV Array : spsPVArrayLib/PV Array  Commented=on  Npar=5  Nser=14  PlotType=array @ 1000 W/m2 & specified temperatures  S_vec=[ 1000]  Temp_C_vec=[ 25 ]  ModuleName=Trina Solar TSM-240PA05.30  PlotWhenSelected=off  Pm=239.856  Ncell=60  Voc=37.2  Isc=8.37  Vm=30.4  Im=7.89  beta_Voc_pc=-0.35  alpha_Isc_pc=0.06  beta_Voc=-0.1302  alpha_Isc=0.005022  IL=8.3942  I0=1.9964e-10  nI=0.98701  Rsh=355.1808  Rs=0.28785  RobustModel=off  RobustCellTemperature=313.3991  BAL=on  Tc=1e-6  Tfilter=5e-5
      settings: AttributesFormatString=|
      | %<ModuleName>
      | %<Nser>-module string
      | %<Npar> parallel strings
  PV1 : spsThreePhaseVIMeasurementLib/Three-Phase V-I Measurement  VoltageMeasurement=phase-to-ground  SetLabelV=off  LabelV=Vabc_grid  Vpu=off  VpuLL=off  CurrentMeasurement=yes  SetLabelI=off  LabelI=Iabc_grid  Ipu=off  Pbase=100e6  Vbase=500e3  OutputType=Magnitude  PhasorSimulation=off  PSBequivalent=0
  Power Factor Block1 : Subsystem  mask(Power Factor Block){Freq=50, Vinit=[0, 0], Iinit=[0, 0], Ts=0}
      mask prompts: Freq "Fundamental frequency (Hz):"; Vinit "Voltage initial input [ Mag, Phase (degrees) ]:"; Iinit "Current initial input [ Mag, Phase (degrees) ]:"; Ts "Sample time:"
      mask help:
      | Power Factor Block developed by Dr Rodney Tan
      | Version 1.01 (Aug 2016)
      |
      | Compute power factor and phase angle of AC circuit voltage-current pair at fundamental frequency.
      |
      | The computation is based on Power block and Complex number function block.
      |
      | For the first cycle of simulation, the outputs are held constant to the powers computed for the Voltage initial input and Current initial input parameters.
      mask Help:
      | <b>Fundamental Frequency (Hz)</b>
      | Specify the measurement fundamental frequency, in hertz, of the input signal.
      | 
      | <b>Voltage initial input [ Mag, Phase (degrees) ]</b>
      | Specify the voltage initial magnitude and phase to set a constant output for the first cycle of simulation.
      | 
      | <b>Current initial input [ Mag, Phase (degrees) ]</b>
      | Specify the current initial magnitude and phase to set a constant output for the first cycle of simulation.
      | 
      | <b>Sample Time</b>
      | Specify the sample time of the block, in seconds. Set to 0 to implement a continuous block.
      mask TypeOptions Freq: Power/Freq
      mask TypeOptions Vinit: Power/Vinit
      mask TypeOptions Iinit: Power/Iinit
      mask TypeOptions Ts: Power/Ts
  Product : Product
  Rate Limiter : RateLimiter  Commented=on  RisingSlewLimit=5000  FallingSlewLimit=-5000  SampleTimeMode=inherited  LinearizeAsGain=off
  SSN Interface Block (3ph) : artemis/SSN/Nodal Interface Blocks/SSN Interface Block (3ph)  nb_phase=3  nb_port=2  p1_type=I-type(Left)  p2_type=V-type (Right)  p3_type=V-type(Left)  p4_type=V-type(Left)  p5_type=V-type(Left)  p6_type=V-type(Left)  p7_type=V-type(Left)  p8_type=V-type(Left)  p9_type=V-type(Left)  p10_type=V-type(Left)  p11_type=V-type(Left)  p12_type=V-type(Left)  p13_type=V-type(Left)  p14_type=V-type(Left)  p15_type=V-type(Left)  p16_type=V-type(Left)  I_port_shunt_resistance=1e9
  Scope : Scope  NumInputPorts=3
  Series RLC Branch : spsSeriesRLCBranchLib/Series RLC Branch  LConnTagsString=__new0  RConnTagsString=__new0  BranchType=C  Resistance=1  Inductance=1e-3  SetiL0=off  InitialCurrent=0  Capacitance=C_cc_proj  Setx0=on  InitialVoltage=Vdc  Measurements=None
  Step : Step  Time=0.5  SampleTime=0
  Subsystem : Subsystem
  Subsystem1 : Subsystem
  Switch : Switch  Criteria=u2 > Threshold
  Switch1 : Switch  Criteria=u2 > Threshold
  Terminator{,1..2,4..6} (6 alike) : Terminator
  Three Phase Converter1 : ssn_inverter_model/ARTEMiS SSN IVIC  Arms=3  SnubberResistance=800  SnubberCapacitance=inf  Device=IGBT / Diodes  Ron=Ron  Lon=0  ForwardVoltages=[0.001 0.001]  ForwardVoltage=0  GTOparameters=[ 10e-6 , 20e-6 ]  IGBTparameters=[ 1e-6 , 2e-6 ]*0  Measurements=None  Measurements_2=None  converterType=Rectifier
  Three-Phase Series RLC Load : spsThreePhaseSeriesRLCLoadLib/Three-Phase Series RLC Load  Commented=on  LConnTagsString=A|B|C  Configuration=Y (grounded)  NominalVoltage=227  Vabc=[1e3 1e3 1e3]  Vabcp=[1e3 1e3 1e3]  NominalFrequency=60  UnbalancedPower=off  ActivePower=80e3  InductivePower=15e3  CapacitivePower=0  Pabc=[10e3 9e3 11e3]  QLabc=[100 90 110]  QCabc=[100 90 110]  Pabcp=[10e3 9e3 11e3]  QLabcp=[100 90 110]  QCabcp=[100 90 110]  Measurements=None  LoadType=constant Z
  Three-Phase Breaker : spsThreePhaseBreakerLib/Three-Phase Breaker  InitialState=open  SwitchA=on  SwitchB=on  SwitchC=on  SwitchTimes="[1/60  5/60]"  External=on  BreakerResistance=0.001  SnubberResistance=1e6  SnubberCapacitance=inf  Measurements=None
  VSC_Control : Subsystem
      settings: PortSchema="{\"entries\":[{\"content\":{\"sides\":[{\"content\":{\"connectorIds\":[\"In1\",\"In2\",\"In3\",\"In4\"]},\"type\":\"ConnectorPlacement.EquallySpacedRectSide\",\"uuid\":\"45e52e2a-5d2e-4b01-a357-9d3073978641\"},{\"content\":{\"connectorIds\":[\"Out1\",\"Out2\",\"Out3\"],\"side\":\"RIGHT\"},\"type\":\"ConnectorPlacement.EquallySpacedRectSide\",\"uuid\":\"500a659a-c60e-4c3f-b5c2-04d8fe26286a\"},{\"content\":{\"connectorIds\":[\"In5\",\"In6\"],\"side\":\"TOP\"},\"type\":\"ConnectorPlacement.EquallySpacedRectSide\",\"uuid\":\"e5a9e837-077a-4c9c-b808-725d6018483b\"},{\"content\":{\"connectorIds\":[],\"side\":\"HIDDEN\"},\"type\":\"ConnectorPlacement.EquallySpacedRectSide\",\"uuid\":\"1c877ae8-e0c9-4faf-8b8c-99cd40b797b6\"}]},\"type\":\"ConnectorPlacement.EquallySpacedConnector\",\"uuid\":\"17a691b0-ccba-4cde-88e8-165a3a0c6333\"}],\"packageUris\":[\"http://schema.mathworks.com/mf0/Connector/R2020b\"],\"version\":\"1.0\"}"
  V_to_pu : Gain  Gain=1/(400*sqrt(2)/sqrt(3))  SaturateOnIntegerOverflow=on  OutDataTypeStr=Inherit: Same as input  ParamDataTypeStr=Inherit: Same as input
  V_to_pu1 : Gain  Gain=1/(400*sqrt(2)/sqrt(3))  SaturateOnIntegerOverflow=on  OutDataTypeStr=Inherit: Same as input  ParamDataTypeStr=Inherit: Same as input
  Vmpp1 : Constant  Value=Vdc
  Voltage Measurement : spsVoltageMeasurementLib/Voltage Measurement  PhasorSimulation=off  OutputType=Complex  PSBequivalent=0
  a : PMIOPort  Side=Right
  b : PMIOPort  Port=2  Side=Right
  c : PMIOPort  Port=3  Side=Right
  PV_m : Outport
  wires:
  [Vdc] -> Subsystem1/3(Vdc)  "Vdc"
  [Pca] -> Subsystem1/4(P_PV)  "P_PV"
  [Iabc_PV] -> Subsystem1/1(Iabc)
  [Iabc_PV] -> Subsystem1/2(In2)
  From20/1 -> APC_algorithm/4(Fault)
  PV/1 -> [Vabc_PV]
  [Vdc] -> VSC_Control/3(Vdc_mes)
  Iq_ref1/1 -> VSC_Control/4(Iq_ref)
  Constant7/1 -> APC_algorithm/2(Freq_ref)
  From34/1 -> APC_algorithm/3(Enable)
  Voltage Measurement/1 -> [Vdc]
  Rate Limiter/1 -> PV Array/1
  [Vabc_PV] -> VSC_Control/1(Vabc)
  Subsystem/1(Iabc) -> [Iabc_PV]
  [Iabc_PV] -> VSC_Control/2(Iabc)
  PV Array/1 -> Goto4/1
  VSC_Control/2(Freq) -> [Freq]
  PLL (3ph)1/2 -> Mux/2  "wt_PV"
  [BRK_PV] -> Scope/3
  PLL (3ph)/2 -> Mux/1  "wt_grid"
  Product/1 -> Three Phase Converter1/1
  BRK_PV/1 -> On Delay/1, [BRK_PV], Switch/3
  [BRK_PV] -> Product/1
  Mux/1 -> Scope/1
  [ENB_PV] -> Scope/2
  V_to_pu1/1 -> PLL (3ph)1/1
  V_to_pu/1 -> PLL (3ph)/1
  Vmpp1/1 -> VSC_Control/6(Vdc_ref)
  [Vabc_grid] -> V_to_pu/1
  VSC_Control/3(P_PV) -> Terminator1/1
  PV1/2 -> [Iabc_grid]
  APC_algorithm/1(Vdc_ref) -> Goto12/1
  [Freq] -> Subsystem1/5(Freq)  "Freq"
  [BRK_PV] -> Three-Phase Breaker/1
  From33/1 -> APC_algorithm/1(Freq_m)
  [Vabc_PV] -> V_to_pu1/1
  [ENB_PV] -> VSC_Control/5(ENB_PV)
  Step/1 -> Switch/2
  Pref/1 -> [Pref]
  PV1/1 -> [Vabc_grid]
  Irra/1 -> Rate Limiter/1
  On Delay/1 -> Switch/1
  Subsystem1/1(Out1) -> PV_m/1
  Switch/1 -> [ENB_PV]
  TempC/1 -> PV Array/2
  [Pref] -> Divide/1
  Constant/1 -> Divide/2
  Divide/1 -> Controlled Current Source2/1
  Power Factor Block1/4(Iabc(rms)) -> [Iabc_rms]
  Power Factor Block1/3(n_PV) -> Terminator2/1
  Power Factor Block1/1(P(kW)) -> [Pca]
  Power Factor Block1/9(Pdc) -> [Pdc]
  Power Factor Block1/6(V abc) -> Terminator5/1
  Power Factor Block1/5("PFabc ") -> Terminator4/1
  [Idc] -> Power Factor Block1/4(Idc)
  Power Factor Block1/8(Vabc(rms)) -> [Vabc_rms]
  Power Factor Block1/7(I abc) -> Terminator6/1
  [Iabc_grid] -> Power Factor Block1/2(Iabc)  "Va (V)"
  Power Factor Block1/2(Qabc(kVAr)) -> Terminator/1
  [Vdc] -> Power Factor Block1/3(Vdc)
  [Vabc_grid] -> Power Factor Block1/1(Vabc)  "Va (V)"
  Current Measurement/1 -> [Idc]
  [Vabc_grid] -> Subsystem1/6(Vabc)  "Vabc_grid"
  VSC_Control/1(Uref) -> Switch1/3
  Demux/1 -> Mux2/1
  PWM/1 -> Demux/1
  [cmd_CHIL] -> Switch1/2
  Mux2/1 -> Switch1/1
  Demux/5 -> Mux2/5
  Demux/4 -> Mux2/4
  Demux/6 -> Mux2/6
  Demux/3 -> Mux2/3
  Demux/2 -> Mux2/2
  Switch1/1 -> Product/2
  cmd_CHIL/1 -> [cmd_CHIL]
  [Vdc] -> Chopper/1(Vdc)
  [Iabc_rms] -> Subsystem1/7(In7)
  [Vabc_rms] -> Subsystem1/8(Vabc_rms)
  connections:
  Three Phase Converter1/RConn2 -- Chopper/RConn1 -- Voltage Measurement/LConn2 -- Controlled Current Source2/LConn1 -- Series RLC Branch/RConn1
  Series RLC Branch/LConn1 -- Chopper/LConn1 -- Three Phase Converter1/RConn1 -- Voltage Measurement/LConn1 -- Current Measurement/RConn1
  L4/RConn2 -- L4/RConn1 -- L4/RConn3 -- Ground/LConn1
  220 kVA 227V / 440V/RConn3 -- L1/RConn3 -- L4/LConn3
  L4/LConn1 -- L1/RConn1 -- 220 kVA 227V / 440V/RConn1
  220 kVA 227V / 440V/RConn2 -- L1/RConn2 -- L4/LConn2
  Carga/RConn3 -- Three-Phase Series RLC Load/LConn1
  Three-Phase Breaker/RConn1 -- PV/RConn1
  PV1/RConn1 -- a/RConn1
  L1/LConn1 -- SSN Interface Block (3ph)/RConn1
  PV/LConn2 -- 220 kVA 227V / 440V/LConn2
  PV/LConn1 -- 220 kVA 227V / 440V/LConn1
  Subsystem/RConn2 -- L/LConn2
  Carga/RConn2 -- Three-Phase Series RLC Load/LConn2
  SSN Interface Block (3ph)/LConn3 -- L/RConn3
  Three Phase Converter1/LConn2 -- Subsystem/LConn2
  PV/LConn3 -- 220 kVA 227V / 440V/LConn3
  Subsystem/LConn1 -- Three Phase Converter1/LConn1
  Subsystem/RConn1 -- L/LConn1
  Subsystem/LConn3 -- Three Phase Converter1/LConn3
  Three-Phase Breaker/LConn1 -- PV1/LConn1
  c/RConn1 -- PV1/RConn3
  L1/LConn2 -- SSN Interface Block (3ph)/RConn2
  PV1/RConn2 -- b/RConn1
  Three-Phase Breaker/LConn3 -- PV1/LConn3
  SSN Interface Block (3ph)/LConn2 -- L/RConn2
  Subsystem/RConn3 -- L/LConn3
  L1/LConn3 -- SSN Interface Block (3ph)/RConn3
  Three-Phase Breaker/RConn2 -- PV/RConn2
  L/RConn1 -- SSN Interface Block (3ph)/LConn1
  Three-Phase Breaker/LConn2 -- PV1/LConn2
  Three-Phase Breaker/RConn3 -- PV/RConn3
  Carga/RConn1 -- Three-Phase Series RLC Load/LConn3
  Controlled Current Source2/RConn1 -- Current Measurement/LConn1

== system Solar_Seguidor/SM_mestre1/eHS ==
  signal1 : Inport  PortDimensions=1
  signal2 : Inport  Port=2  PortDimensions=1
  signal3 : Inport  Port=3  PortDimensions=1
  signal4 : Inport  Port=4  PortDimensions=1
  signal5 : Inport  Port=5  PortDimensions=1
  signal6 : Inport  Port=6  PortDimensions=1
  signal7 : Inport  Port=7  PortDimensions=1
  OpOutput_parameter_set_id : rtlab/OpOutput  identifier_use=parameter_set_id  identifier_hide=eHS/parameter_set_id  nb_parents_identifier=1
      settings: SourceProductName=RT-LAB
  OpOutput_signal1 : rtlab/OpOutput  identifier_use=signal1  identifier_hide=eHS/signal1  nb_parents_identifier=1
      settings: SourceProductName=RT-LAB
  OpOutput_signal2 : rtlab/OpOutput  identifier_use=signal2  identifier_hide=eHS/signal2  nb_parents_identifier=1
      settings: SourceProductName=RT-LAB
  OpOutput_signal3 : rtlab/OpOutput  identifier_use=signal3  identifier_hide=eHS/signal3  nb_parents_identifier=1
      settings: SourceProductName=RT-LAB
  OpOutput_signal4 : rtlab/OpOutput  identifier_use=signal4  identifier_hide=eHS/signal4  nb_parents_identifier=1
      settings: SourceProductName=RT-LAB
  OpOutput_signal5 : rtlab/OpOutput  identifier_use=signal5  identifier_hide=eHS/signal5  nb_parents_identifier=1
      settings: SourceProductName=RT-LAB
  OpOutput_signal6 : rtlab/OpOutput  identifier_use=signal6  identifier_hide=eHS/signal6  nb_parents_identifier=1
      settings: SourceProductName=RT-LAB
  OpOutput_signal7 : rtlab/OpOutput  identifier_use=signal7  identifier_hide=eHS/signal7  nb_parents_identifier=1
      settings: SourceProductName=RT-LAB
  internal : Constant  Value=0
  internal_or_external : Constant  Value=0
  parameter_set_switch : Switch  Criteria=u2 > Threshold
  wires:
  signal1/1 -> OpOutput_signal1/1
  signal2/1 -> OpOutput_signal2/1
  signal3/1 -> OpOutput_signal3/1
  signal4/1 -> OpOutput_signal4/1
  signal5/1 -> OpOutput_signal5/1
  signal6/1 -> OpOutput_signal6/1
  signal7/1 -> OpOutput_signal7/1
  internal_or_external/1 -> parameter_set_switch/2
  internal/1 -> parameter_set_switch/3
  parameter_set_switch/1 -> OpOutput_parameter_set_id/1

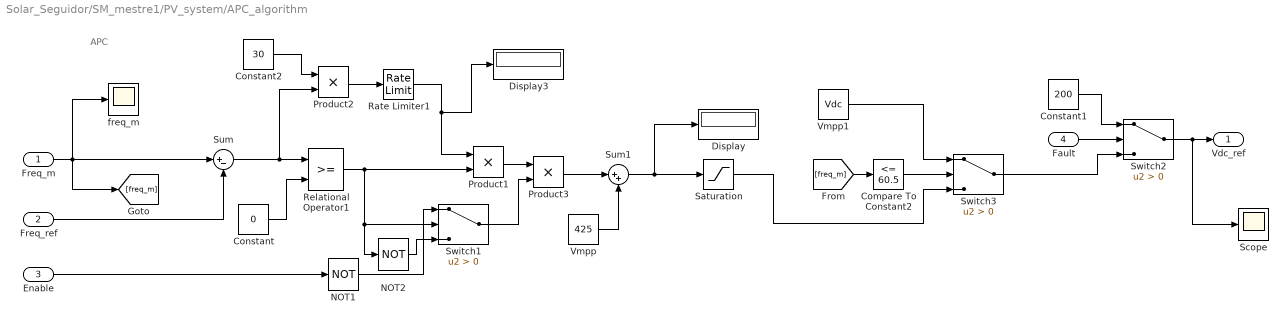
== system Solar_Seguidor/SM_mestre1/PV_system/APC_algorithm ==
  note: APC
  Freq_m : Inport
  Freq_ref : Inport  Port=2
  Enable : Inport  Port=3
  Fault : Inport  Port=4
  Compare To Constant2 : simulink/Logic and Bit Operations/Compare To Constant  relop=<=  const=60.5  OutDataTypeStr=boolean
  Constant : Constant  Value=0
  Constant1 : Constant  Value=200
  Constant2 : Constant  Value=30
  Display : Display
  Display3 : Display
  NOT1 : Logic  Operator=NOT  IconShape=distinctive  AllPortsSameDT=off  OutDataTypeStr=boolean
  NOT2 : Logic  Operator=NOT  IconShape=distinctive  AllPortsSameDT=off  OutDataTypeStr=boolean
  Product1 : Product
  Product2 : Product
  Product3 : Product
  Rate Limiter1 : RateLimiter  RisingSlewLimit=200  FallingSlewLimit=-200  SampleTimeMode=inherited
  Relational Operator1 : RelationalOperator  OutDataTypeStr=boolean  RndMeth=Simplest
  Saturation : Saturate  UpperLimit=580  LowerLimit=0
  Scope : Scope
  Sum : Sum  Inputs=|+-
  Sum1 : Sum  Inputs=|++
  Switch1 : Switch  Criteria=u2 > Threshold
  Switch2 : Switch  Criteria=u2 > Threshold
  Switch3 : Switch  Criteria=u2 > Threshold
  Vmpp : Constant  Value=425
  Vmpp1 : Constant  Value=Vdc
  freq_m : Scope
  Vdc_ref : Outport
  wires:
  Product3/1 -> Sum1/1
  Sum1/1 -> Saturation/1, Display/1
  Product1/1 -> Product3/1
  Sum/1 -> Product2/2, Relational Operator1/1
  Switch1/1 -> Product3/2
  Relational Operator1/1 -> NOT2/1, Switch1/2, Product1/2
  NOT2/1 -> Switch1/3
  Constant2/1 -> Product2/1
  Product2/1 -> Rate Limiter1/1
  Rate Limiter1/1 -> Display3/1, Product1/1
  Enable/1 -> NOT1/1
  Vmpp/1 -> Sum1/2
  Constant/1 -> Relational Operator1/2
  Freq_m/1 -> freq_m/1, Sum/1, [freq_m]
  NOT1/1 -> Switch1/1
  Freq_ref/1 -> Sum/2
  Switch2/1 -> Scope/1, Vdc_ref/1
  Fault/1 -> Switch2/2
  Constant1/1 -> Switch2/1
  [freq_m] -> Compare To Constant2/1
  Compare To Constant2/1 -> Switch3/2
  Saturation/1 -> Switch3/3
  Vmpp1/1 -> Switch3/1
  Switch3/1 -> Switch2/3
